simulink model "aurora_cpu_ch0_ver2_rtxsg"  (R2019b)
settings: Solver=ode45  StartTime=0.0  StopTime=1/6000  RelTol=1e-3  EnableMultiTasking=on
PreLoadFcn:
  | period=5e-9;
InitFcn:
  | period=5e-9;
undefined symbols (not defined in the file): DUALSFP, EX, opGetFPGAPeriod, VC707_2
libraries: xbsIndex_r4 x170, rtxsg_tools x22, rtxsg_communication x3, rtxsg_common x3, HighSpeedCommIO_lib x2, rtxsg_serdes_lib x2, vc707_lib x1
(part 1 of 4)
PreSaveFcn:
  | try, efsUpdateVersionAnnotation, end
settings Model: Creator=SebastienCense  LastModifiedBy=nei
settings SolverCC: AutoInsertRateTranBlk=on
settings DataIOCC: LimitDataPoints=on  SaveFormat=Array  SignalLoggingSaveFormat=ModelDataLogs  ReturnWorkspaceOutputs=off
settings OptimizationCC: ExpressionDepthLimit=2147483647  LifeSpan=inf
settings DebuggingCC: UnderspecifiedInitializationDetection=Classic  MergeDetectMultiDrivingBlocksExec=none  SolverPrmCheckMsg=warning  FcnCallInpInsideContextMsg=warning  StateNameClashWarn=warning  SFUnexpectedBacktrackingDiag=warning  SFNoUnconditionalDefaultTransitionDiag=warning  SFExecutionAtInitializationDiag=none  ArithmeticOperatorsInVariantConditions=warning
settings HardwareCC: ProdBitPerPointer=32  ProdBitPerSizeT=32  ProdBitPerPtrDiffT=32  ProdLargestAtomicFloat=None  ProdIntDivRoundTo=Undefined  ProdEndianess=Unspecified  ProdWordSize=32  ProdHWDeviceType=32-bit Generic
settings ModelReferenceCC: PropagateSignalLabelsOutOfModel=off
settings SFSimCC: SimUseLocalCustomCode=off  CustomCodeUndefinedFunction=UseInterfaceOnly
settings RTWCC: RTWUseLocalCustomCode=off
settings CodeAppCC: StateflowObjectComments=on
settings GRTTargetCC: TargetLangStandard=C89/C90 (ANSI)  GeneratePreprocessorConditionals=Disable all  CombineOutputUpdateFcns=off  GRTInterface=on
settings ConfigComp: CovMetricSettings=dw  CovHtmlReporting=on  CovSaveCumulativeToWorkspaceVar=on  CovSaveSingleToWorkspaceVar=on  CovExternalEMLEnable=off  CovSFcnEnable=off

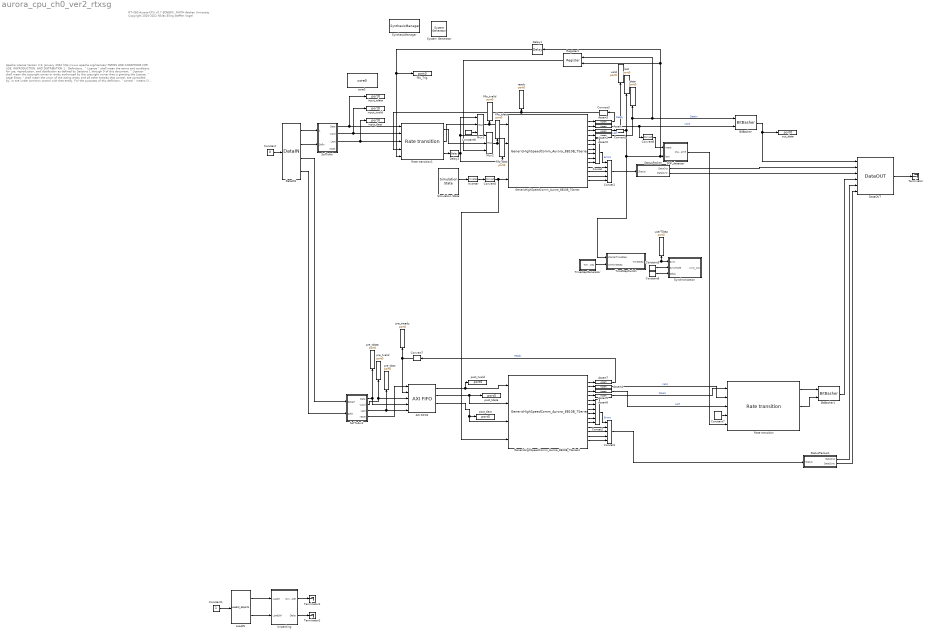
== system aurora_cpu_ch0_ver2_rtxsg ==
  note: RT-XSG Aurora-CPU v0.7
      | EONERC, RWTH Aachen University
      | Copyright 2020-2022
      | Niklas Eiling
      | Steffen Vogel
  note: Apache License
      | Version 2.0, January 2004
      | http://www.apache.org/licenses/
      | TERMS AND CONDITIONS FOR USE, REPRODUCTION, AND DISTRIBUTION
      | 1 . Definitions .
      | " License " shall mean the terms and conditions for use, reproduction, and distribution as defined by Sections 1 through 9 of this document.
      | " Licensor " shall mean the copyright owner or entity authorized by the copyright owner that is granting the License.
      | " Legal Entity " shall mean the union of the acting entity and all other entities that control, are controlled by, or are under common control with that entity. For the purposes of this definition, " control " means (i) the power, direct or indirect, to cause the direction or management of such entity, whether by contract or otherwise, or (ii) ownership of fifty percent (50%) or more of the outstanding shares, or (iii) beneficial ownership of such entity.
      | " You " (or " Your ") shall mean an individual or Legal Entity exercising permissions granted by this License.
      | " Source " form shall mean the preferred form for making modifications, including but not limited to software source code, documentation source, and configuration files.
      | " Object " form shall mean any form resulting from mechanical transformation or translation of a Source form, including but not limited to compiled object code, generated documentation, and conversions to other media types.
      | " Work " shall mean the work of authorship, whether in Source or Object form, made available under the License, as indicated by a copyright notice that is included in or attached to the work (an example is provided in the Appendix below).
      | " Derivative Works " shall mean any work, whether in Source or Object form, that is based on (or derived from) the Work and for which the editorial revisions, annotations, elaborations, or other modifications represent, as a whole, an original work of authorship. For the purposes of this License, Derivative Works shall not include works that remain separable from, or merely link (or bind by name) to the interfaces of, the Work and Derivative Works thereof.
      | " Contribution " shall mean any work of authorship, including the original version of the Work and any modifications or additions to that Work or Derivative Works thereof, that is intentionally submitted to Licensor for inclusion in the Work by the copyright owner or by an individual or Legal Entity authorized to submit on behalf of the copyright owner. For the purposes of this definition, " submitted " means any form of electronic, verbal, or written communication sent to the Licensor or its representatives, including but not limited to communication on electronic mailing lists, source code control systems, and issue tracking systems that are managed by, or on behalf of, the Licensor for the purpose of discussing and improving the Work, but excluding communication that is conspicuously marked or otherwise designated in writing by the copyright owner as " Not a Contribution. "
      | " Contributor " shall mean Licensor and any individual or Legal Entity on behalf of whom a Contribution has been received by Licensor and subsequently incorporated within the Work.
      | 2 . Grant of Copyright License . Subject to the terms and conditions of this License, each Contributor hereby grants to You a perpetual, worldwide, non-exclusive, no-charge, royalty-free, irrevocable copyright license to reproduce, prepare Derivative Works of, publicly display, publicly perform, sublicense, and distribute the Work and such Derivative Works in Source or Object form.
      | 3 . Grant of Patent License . Subject to the terms and conditions of this License, each Contributor hereby grants to You a perpetual, worldwide, non-exclusive, no-charge, royalty-free, irrevocable (except as stated in this section) patent license to make, have made, use, offer to sell, sell, import, and otherwise transfer the Work, where such license applies only to those patent claims licensable by such Contributor that are necessarily infringed by their Contribution(s) alone or by combination of their Contribution(s) with the Work to which such Contribution(s) was submitted. If You institute patent litigation against any entity (including a cross-claim or counterclaim in a lawsuit) alleging that the Work or a Contribution incorporated within the Work constitutes direct or contributory patent infringement, then any patent licenses granted to You under this License for that Work shall terminate as of the date such litigation is filed.
      | 4 . Redistribution . You may reproduce and distribute copies of the Work or Derivative Works thereof in any medium, with or without modifications, and in Source or Object form, provided that You meet the following conditions:
      | You must give any other recipients of the Work or Derivative Works a copy of this License; and
      | You must cause any modified files to carry prominent notices stating that You changed the files; and
      | You must retain, in the Source form of any Derivative Works that You distribute, all copyright, patent, trademark, and attribution notices from the Source form of the Work, excluding those notices that do not pertain to any part of the Derivative Works; and
      | If the Work includes a " NOTICE " text file as part of its distribution, then any Derivative Works that You distribute must include a readable copy of the attribution notices contained within such NOTICE file, excluding those notices that do not pertain to any part of the Derivative Works, in at least one of the following places: within a NOTICE text file distributed as part of the Derivative Works; within the Source form or documentation, if provided along with the Derivative Works; or, within a display generated by the Derivative Works, if and wherever such third-party notices normally appear. The contents of the NOTICE file are for informational purposes only and do not modify the License. You may add Your own attribution notices within Derivative Works that You distribute, alongside or as an addendum to the NOTICE text from the Work, provided that such additional attribution notices cannot be construed as modifying the License.
      |
      | You may add Your own copyright statement to Your modifications and may provide additional or different license terms and conditions for use, reproduction, or distribution of Your modifications, or for any such Derivative Works as a whole, provided Your use, reproduction, and distribution of the Work otherwise complies with the conditions stated in this License.
      | 5 . Submission of Contributions . Unless You explicitly state otherwise, any Contribution intentionally submitted for inclusion in the Work by You to the Licensor shall be under the terms and conditions of this License, without any additional terms or conditions. Notwithstanding the above, nothing herein shall supersede or modify the terms of any separate license agreement you may have executed with Licensor regarding such Contributions.
      | 6 . Trademarks . This License does not grant permission to use the trade names, trademarks, service marks, or product names of the Licensor, except as required for reasonable and customary use in describing the origin of the Work and reproducing the content of the NOTICE file.
      | 7 . Disclaimer of Warranty . Unless required by applicable law or agreed to in writing, Licensor provides the Work (and each Contributor provides its Contributions) on an "AS IS" BASIS, WITHOUT WARRANTIES OR CONDITIONS OF ANY KIND, either express or implied, including, without limitation, any warranties or conditions of TITLE, NON-INFRINGEMENT, MERCHANTABILITY, or FITNESS FOR A PARTICULAR PURPOSE. You are solely responsible for determining the appropriateness of using or redistributing the Work and assume any risks associated with Your exercise of permissions under this License.
      | 8 . Limitation of Liability . In no event and under no legal theory, whether in tort (including negligence), contract, or otherwise, unless required by applicable law (such as deliberate and grossly negligent acts) or agreed to in writing, shall any Contributor be liable to You for damages, including any direct, indirect, special, incidental, or consequential damages of any character arising as a result of this License or out of the use or inability to use the Work (including but not limited to damages for loss of goodwill, work stoppage, computer failure or malfunction, or any and all other commercial damages or losses), even if such Contributor has been advised of the possibility of such damages.
      | 9 . Accepting Warranty or Additional Liability . While redistributing the Work or Derivative Works thereof, You may choose to offer, and charge a fee for, acceptance of support, warranty, indemnity, or other liability obligations and/or rights consistent with this License. However, in accepting such obligations, You may act only on Your own behalf and on Your sole responsibility, not on behalf of any other Contributor, and only if You agree to indemnify, defend, and hold each Contributor harmless for any liability incurred by, or claims asserted against, such Contributor by reason of your accepting any such warranty or additional liability.
      | END OF TERMS AND CONDITIONS
  " System Generator" : xbsIndex_r4/ System Generator  Tag=genX  xilinxfamily=virtex7  part=xc7vx485t  speed=-2  package=ffg1761  synthesis_tool=Vivado  clock_wrapper=Clock Enables  directory=./netlist  proj_type=Vivado  Synth_file=Vivado Synthesis Defaults  Impl_file=Vivado Implementation Defaults  testbench=off  simulink_period=1e-8  sysclk_period=5  dcm_input_clock_period=10  incr_netlist=off  trim_vbits=Everywhere in SubSystem  dbl_ovrd=According to Block Masks  core_generation=According to Block Masks  run_coregen=off  deprecated_control=off  eval_field=0  block_type=sysgen
  AXI FIFO1 : xbsIndex_r4/AXI FIFO  input_depth_axis=128  actual_fifo_depth_label=130  enable_tdata=on  enable_tdest=off  enable_tstrb=off  enable_tready=on  enable_tid=off  enable_tuser=off  enable_tkeep=off  enable_tlast=on  has_aresetn=on  enable_data_counts_axis=off  fifo_implementation_type_axis=Common Clock Block RAM  trim_axipin_name=on  programmable_full_type_axis=Full  full_threshold_assert_value_axis=0  programmable_empty_type_axis=Empty  empty_threshold_assert_value_axis=1022  underflow_flag_axi=0  underflow_sense_axi=Active High  overflow_flag_axi=0  overflow_sense_axi=Active High  block_type=axi_fifo
  Assert{,3..4,7} (4 alike) : xbsIndex_r4/Assert  assert_type=off  type_source=Explicitly  gui_display_data_type=Fixed-point  arith_type="Signed  (2's comp)"  n_bits=16  bin_pt=14  preci_type=Single  exp_width=8  frac_width=24  assert_rate=on  rate_source=Explicitly  period=opGetFPGAPeriod(bdroot)  output_port=on  block_type=assert
  Assert{1..2,5..6} (4 alike) : xbsIndex_r4/Assert  assert_type=off  type_source=Explicitly  gui_display_data_type=Boolean  arith_type=Boolean  n_bits=16  bin_pt=14  preci_type=Single  exp_width=8  frac_width=24  assert_rate=on  rate_source=Explicitly  period=opGetFPGAPeriod(bdroot)  output_port=on  block_type=assert
  BitBasher : xbsIndex_r4/BitBasher  bitexpr=DataOut={WE,Data}  display_expr=off  sr_1=DataOut  arith_type1=Unsigned  bin_pt1=0  sr_2=2  arith_type2=Unsigned  bin_pt2=0  sr_3=3  arith_type3=Unsigned  bin_pt3=0  sr_4=4  arith_type4=Unsigned  bin_pt4=0  dbl_ovrd=off  block_type=bitbasher
  BitBasher1 : xbsIndex_r4/BitBasher  bitexpr=DataOut={WE,Data}  display_expr=off  sr_1=DataOut  arith_type1=Unsigned  bin_pt1=0  sr_2=2  arith_type2=Unsigned  bin_pt2=0  sr_3=3  arith_type3=Unsigned  bin_pt3=0  sr_4=4  arith_type4=Unsigned  bin_pt4=0  dbl_ovrd=off  block_type=bitbasher
  Concat : xbsIndex_r4/Concat  num_inputs=6  dbl_ovrd=off  block_type=concat
  Concat1 : xbsIndex_r4/Concat  num_inputs=5  dbl_ovrd=off  block_type=concat
  Concat2 : xbsIndex_r4/Concat  num_inputs=6  dbl_ovrd=off  block_type=concat
  Concat3 : xbsIndex_r4/Concat  num_inputs=5  dbl_ovrd=off  block_type=concat
  Constant : Constant  Value=0
  Constant1 : Constant
  Constant5 : xbsIndex_r4/Constant  const=0  gui_display_data_type=Fixed-point  arith_type=Unsigned  n_bits=2  bin_pt=0  preci_type=Single  exp_width=8  frac_width=24  explicit_period=on  period=opGetFPGAPeriod(bdroot)  equ=P=C  opselect=C  inp2=PCIN>>17  opr=+  inp1=P  carry=CIN  dbl_ovrd=off  block_type=constant
  Constant6 : xbsIndex_r4/Constant  const=0  gui_display_data_type=Fixed-point  arith_type=Unsigned  n_bits=22  bin_pt=0  preci_type=Single  exp_width=8  frac_width=24  explicit_period=on  period=opGetFPGAPeriod(bdroot)  equ=P=C  opselect=C  inp2=PCIN>>17  opr=+  inp1=P  carry=CIN  dbl_ovrd=off  block_type=constant
  Constant7 : xbsIndex_r4/Constant  const=1  gui_display_data_type=Boolean  arith_type=Boolean  n_bits=1  bin_pt=0  preci_type=Single  exp_width=8  frac_width=24  explicit_period=on  period=opGetFPGAPeriod(bdroot)  equ=P=C  opselect=C  inp2=PCIN>>17  opr=+  inp1=P  carry=CIN  dbl_ovrd=off  block_type=constant
  Constant8 : xbsIndex_r4/Constant  const=1  gui_display_data_type=Boolean  arith_type=Boolean  n_bits=1  bin_pt=0  preci_type=Single  exp_width=8  frac_width=24  explicit_period=off  period=1  equ=P=C  opselect=C  inp2=PCIN>>17  opr=+  inp1=P  carry=CIN  dbl_ovrd=off  block_type=constant
  Convert1 : xbsIndex_r4/Convert  gui_display_data_type=Boolean  arith_type=Boolean  n_bits=1  bin_pt=0  float_type=Single  exp_bits=8  fraction_bits=24  quantization=Truncate  overflow=Wrap  en=off  latency=0  pipeline=off  dbl_ovrd=off  block_type=convert
  Convert3 : xbsIndex_r4/Convert  gui_display_data_type=Boolean  arith_type=Boolean  n_bits=16  bin_pt=14  float_type=Single  exp_bits=8  fraction_bits=24  quantization=Truncate  overflow=Wrap  en=off  latency=0  pipeline=off  dbl_ovrd=off  block_type=convert
  Convert5 : xbsIndex_r4/Convert  gui_display_data_type=Boolean  arith_type=Boolean  n_bits=1  bin_pt=0  float_type=Single  exp_bits=8  fraction_bits=24  quantization=Truncate  overflow=Wrap  en=off  latency=0  pipeline=off  dbl_ovrd=off  block_type=convert
  Convert7 : xbsIndex_r4/Convert  gui_display_data_type=Boolean  arith_type=Boolean  n_bits=16  bin_pt=14  float_type=Single  exp_bits=8  fraction_bits=24  quantization=Truncate  overflow=Wrap  en=off  latency=0  pipeline=off  dbl_ovrd=off  block_type=convert
  Convert8 : xbsIndex_r4/Convert  gui_display_data_type=Boolean  arith_type=Boolean  n_bits=1  bin_pt=0  float_type=Single  exp_bits=8  fraction_bits=24  quantization=Truncate  overflow=Wrap  en=off  latency=0  pipeline=off  dbl_ovrd=off  block_type=convert
  DataIN1 : rtxsg_communication/DataIN  NbPorts=2  trans_mode=11  sof_mode=11  DataProtect=00  trans_mode2=0  sof_mode2=0  DataProtect2=0  clk_period=opGetFPGAPeriod(bdroot)  MaxNbPorts=64  AlignOn=off  DataPort1ProtectValue=0  DataPort2ProtectValue=0  DataPort3ProtectValue=0  DataPort4ProtectValue=0  DataPort5ProtectValue=0  DataPort6ProtectValue=0  DataPort7ProtectValue=0  DataPort8ProtectValue=0  DataPort9ProtectValue=0  DataPort10ProtectValue=0  DataPort11ProtectValue=0  DataPort12ProtectValue=0  DataPort13ProtectValue=0  DataPort14ProtectValue=0  DataPort15ProtectValue=0  DataPort16ProtectValue=0  DataPort17ProtectValue=0  DataPort18ProtectValue=0  DataPort19ProtectValue=0  DataPort20ProtectValue=0  DataPort21ProtectValue=0  DataPort22ProtectValue=0  DataPort23ProtectValue=0  DataPort24ProtectValue=0  DataPort25ProtectValue=0  DataPort26ProtectValue=0  DataPort27ProtectValue=0  DataPort28ProtectValue=0  DataPort29ProtectValue=0  DataPort30ProtectValue=0  DataPort31ProtectValue=0  DataPort32ProtectValue=0  DataPort33ProtectValue=0  DataPort34ProtectValue=0  DataPort35ProtectValue=0  DataPort36ProtectValue=0  DataPort37ProtectValue=0  DataPort38ProtectValue=0  DataPort39ProtectValue=0  DataPort40ProtectValue=0  DataPort41ProtectValue=0  DataPort42ProtectValue=0  DataPort43ProtectValue=0  DataPort44ProtectValue=0  DataPort45ProtectValue=0  DataPort46ProtectValue=0  DataPort47ProtectValue=0  DataPort48ProtectValue=0  DataPort49ProtectValue=0  DataPort50ProtectValue=0  DataPort51ProtectValue=0  DataPort52ProtectValue=0  DataPort53ProtectValue=0  DataPort54ProtectValue=0  DataPort55ProtectValue=0  DataPort56ProtectValue=0  DataPort57ProtectValue=0  DataPort58ProtectValue=0  DataPort59ProtectValue=0  DataPort60ProtectValue=0  DataPort61ProtectValue=0  DataPort62ProtectValue=0  DataPort63ProtectValue=0  DataPort64ProtectValue=0
  DataOUT : rtxsg_communication/DataOUT  NbPorts=4  buf_type=1111  ExtSync=1010  buf_type2=0  ExtSync2=0  autosendport=0000000000000000  autosendlength=4  clk_period=opGetFPGAPeriod(bdroot)  MaxNbPorts=64  UseOldImplementation=false
  Delay1 : xbsIndex_r4/Delay  rst=off  infoeditControl=Selection of Reset will increase slice count due to use of real FFs and instead of SRLs  en=off  latency=1  reg_retiming=off  dbl_ovrd=off  block_type=delay
  Delay3 : xbsIndex_r4/Delay  rst=off  infoeditControl=Selection of Reset will increase slice count due to use of real FFs and instead of SRLs  en=off  latency=1  reg_retiming=off  dbl_ovrd=off  block_type=delay
  GenericHighSpeedComm_Aurora_8B10B_7Series : HighSpeedCommIO_lib/GenericHighSpeedComm_Aurora_8B10B_7Series  ChannelNumber=Channel 0  MGTRefClkFrequency=250 MHz  Protocol=Aurora 8B10B  LineRate=2 Gbps  fifoOverflowErrorPortOn=off  StatusPortOn=on  StatisticPortOn=on  GtResetPortOn=on  RXLastDataPortOn=on  DisableCRCOn=on  CRCTestPortOn=off  endianSelect=Big Endian  clk_period=opGetFPGAPeriod(bdroot)  Technology=7Series  ExtClkXCoord=0  ExtClkYCoord=0  CPLLREFCLKSEL=001  QPLLREFCLKSEL=001  TXDIFFCTRL=1000 (0.807 mVppd)  TXPRECURSOR=00111 (1.67 dB)  TXPOSTCURSOR=00011 (0.68 dB)  InterFPGAMode=false  GUI_opened=off
  GenericHighSpeedComm_Aurora_8B10B_7Series1 : HighSpeedCommIO_lib/GenericHighSpeedComm_Aurora_8B10B_7Series  ChannelNumber=Channel 1  MGTRefClkFrequency=250 MHz  Protocol=Aurora 8B10B  LineRate=2 Gbps  fifoOverflowErrorPortOn=off  StatusPortOn=on  StatisticPortOn=on  GtResetPortOn=on  RXLastDataPortOn=on  DisableCRCOn=on  CRCTestPortOn=off  endianSelect=Big Endian  clk_period=opGetFPGAPeriod(bdroot)  Technology=7Series  ExtClkXCoord=0  ExtClkYCoord=0  CPLLREFCLKSEL=001  QPLLREFCLKSEL=001  TXDIFFCTRL=1000 (0.807 mVppd)  TXPRECURSOR=00111 (1.67 dB)  TXPOSTCURSOR=00011 (0.68 dB)  InterFPGAMode=false  GUI_opened=off
  Inverter : xbsIndex_r4/Inverter  en=off  latency=0  dbl_ovrd=off  block_type=inv
  LoadIN : rtxsg_communication/LoadIN_32ports  NbPorts=1  trans_mode=1  trans_mode2=0  clk_period=opGetFPGAPeriod(bdroot)  MaxNbPorts=32  sof_mode=1  sof_mode2=0  AlignOn=off
  Mux1 : xbsIndex_r4/Mux  inputs=2  en=off  latency=0  precision=Full  arith_type=Unsigned  n_bits=16  bin_pt=14  quantization=Truncate  overflow=Wrap  dbl_ovrd=off  block_type=mux
  Mux2 : xbsIndex_r4/Mux  inputs=2  en=off  latency=0  precision=Full  arith_type=Unsigned  n_bits=16  bin_pt=14  quantization=Truncate  overflow=Wrap  dbl_ovrd=off  block_type=mux
  Rate transition : rtxsg_serdes_lib/Rate transition  RXType=AXI (Data/Valid/Last)  NbDataOutputEn=off
      settings: SourceProductName=RT-XSG
  Rate transition1 : rtxsg_serdes_lib/Rate transition  RXType=AXI (Data/Valid/Last)  NbDataOutputEn=off
      settings: SourceProductName=RT-XSG
  Register1 : xbsIndex_r4/Register  init=0  rst=off  en=on  dbl_ovrd=off  block_type=register
  SOF_detector : Subsystem
  Simulation State : rtxsg_common/Simulation State  TimerWidth=22
      settings: SourceProductName=RT-XSG
  SofToAxi : Subsystem
  SofToAxi1 : Subsystem
  StatusPacker : Subsystem
  StatusPacker1 : Subsystem
  Synchronization : Subsystem
  SynthesisManager : rtxsg_tools/SynthesisManager  AllowSave=off  BoardName=Xilinx VC707 development board (Virtex-7 XC7VX485T device) for OP5607 System  RebuildOptions=Always  FPGAVendor=xilinx  FPGAFamily=virtex2p  FPGAModel=xc2vp7  FPGASpeed=-5  FPGAPackage=ff672  clk_period=1e-08  CompilationNames=VC707_2-EX-0001-3_2_10_45-DUALSFP-02-23.bin  ClkFreqIndex=1  opt_resources=0  SecondaryFPGASlot=16  IPCache=0  genBitstream=1  genCfg=0  HSLArchType=1  advanceGeneration=0  HSLLineRate=1
